simulink model "orbital_speed"  (R2025a)
settings: Solver=VariableStepAuto  StartTime=0.0  StopTime=5000.0  RelTol=1e-3

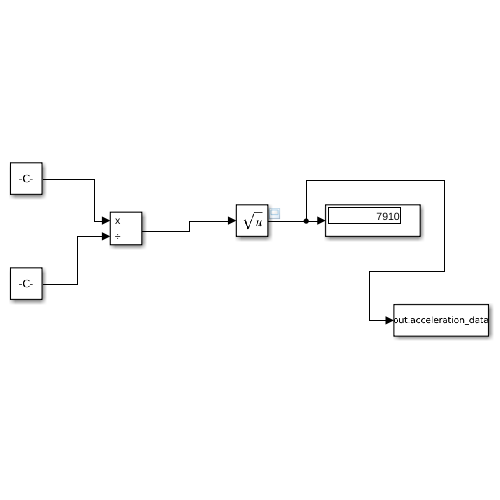
[thumbnail: Simulink's stored preview of the top-level diagram]
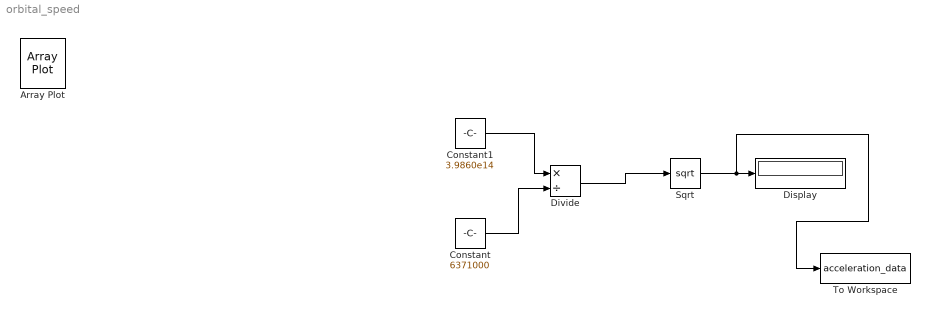
== system orbital_speed ==
  Constant : Constant  Value=6371000
  Constant1 : Constant  Value=3.9860e14
  Display : Display
  Divide : Product  Inputs=*/
  Sqrt : Sqrt
  To Workspace : ToWorkspace  VariableName=acceleration_data  SampleTime=-1
  Array Plot : ArrayPlot  IOType=viewer  IsFloating=on  Visible=on  ContainerLayout="{\"WindowBounds\":[1,1446,1519,682]}"  YLimits=[6921.0645 8898.5115]  DefaultConfigurationName=dsp.scopes.ArrayPlotBlockSpecification
  wires:
  Constant/1 -> Divide/2
  Constant1/1 -> Divide/1
  Divide/1 -> Sqrt/1
  Sqrt/1 -> To Workspace/1, Display/1
